simulink model "Gierwinkel_Schwimmwinkel_zu_Koordinaten"  (R2020b)
settings: Solver=FixedStepAuto  StartTime=simin_radius.time(1,1)  StopTime=simin_radius.time(end,1)-0.01  FixedStep=0.01  RelTol=1e-3
settings Model: PacingRate=32  Creator=Laptop 11  LastModifiedBy=Laptop 11
settings DataIOCC: SaveFormat=Array  ReturnWorkspaceOutputs=off

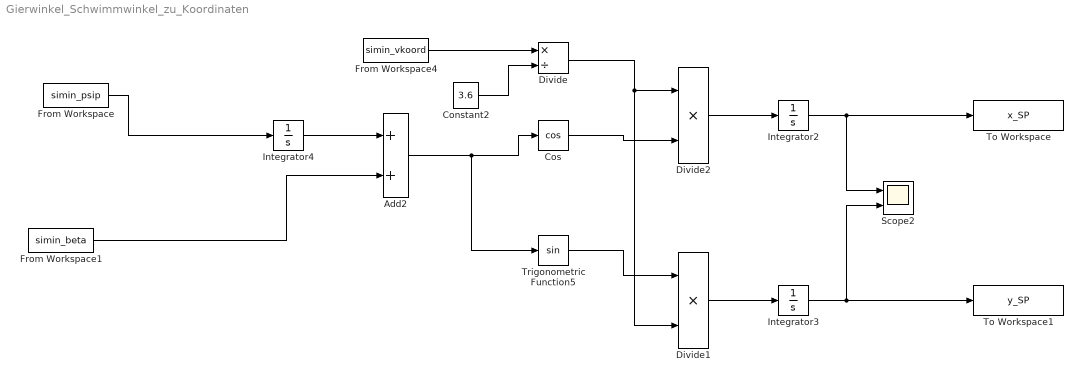
== system Gierwinkel_Schwimmwinkel_zu_Koordinaten ==
  Add2 : Sum
  Constant2 : Constant  Value=3.6
  Cos : Trigonometry  Operator=cos
  Divide : Product  Inputs=*/
  Divide1 : Product  Inputs=**
  Divide2 : Product  Inputs=**
  From Workspace : FromWorkspace  VariableName=simin_psip  ZeroCross=off  OutputAfterFinalValue=Setting to zero
  From Workspace1 : FromWorkspace  VariableName=simin_beta  OutputAfterFinalValue=Setting to zero
  From Workspace4 : FromWorkspace  VariableName=simin_vkoord  OutputAfterFinalValue=Setting to zero
  Integrator2 : Integrator
  Integrator3 : Integrator
  Integrator4 : Integrator
  Scope2 : Scope  NumInputPorts=2
  To Workspace : ToWorkspace  VariableName=x_SP  SaveFormat=Structure  SampleTime=-1
  To Workspace1 : ToWorkspace  VariableName=y_SP  SaveFormat=Structure  SampleTime=-1
  Trigonometric Function5 : Trigonometry
  wires:
  Add2/1 -> Trigonometric Function5/1, Cos/1
  Cos/1 -> Divide2/2
  Trigonometric Function5/1 -> Divide1/1
  Divide2/1 -> Integrator2/1
  Divide1/1 -> Integrator3/1
  Integrator3/1 -> Scope2/2, To Workspace1/1
  Integrator2/1 -> Scope2/1, To Workspace/1
  Integrator4/1 -> Add2/1
  From Workspace/1 -> Integrator4/1
  From Workspace1/1 -> Add2/2
  From Workspace4/1 -> Divide/1
  Constant2/1 -> Divide/2
  Divide/1 -> Divide1/2, Divide2/1
